simulink model "Locomotive_model"  (R2021a)
settings: Solver=ode23s  StartTime=0.0  StopTime=400  RelTol=1e-3
values from neighbouring files (symbols this model uses):
  B = T_friction/omega_b    (= 27.8481991909)    [Train_script.m]
  d = 1250*10^-3    (= 1.25)    [Train_script.m]
  I_motor = Pe_tot/sqrt(3)/V_motor/cos_fi    [Train_script.m]
  id_ref = psi_rd_ref./M    [Train_script.m]
  J = mass_tot*v_max^2/omega_max^2    (= 15228.5481732)    [Train_script.m]
  kp_O = par_reg_speed.Kp    [Train_script.m]
  kp_psi = par_reg_speed.Kp    [Train_script.m]
  kp_s = par_regi.Kp    [Train_script.m]
  Lks = X_lock_eq/(2*pi*50)    [Train_script.m]
  M = (X_noload_eq)/(2*pi*50)    [Train_script.m]
  mass_tot = 89*10^3+11*47*10^3+45*80+45*15    (= 610275)    [Train_script.m]
  pp = 2    [Train_script.m]
  psi_r_max = V_motor*sqrt(3)*0.8/(omega_b*pp)    [Train_script.m]
  psi_rd_ref = traction(:,2).*d/2.*tr./k    [Train_script.m]
  Rks = Rs_eq+Rr_eq    [Train_script.m]
  Rr_eq = Rr*Z    [Train_script.m]
  Rs_eq = Rs*Z    [Train_script.m]
  speed_ref = traction(:,1)    [Train_script.m]
  Ti_O = kp_O/ki_O    [Train_script.m]
  Ti_psi = kp_psi/ki_psi    [Train_script.m]
  Ti_s = kp_s/ki_s    [Train_script.m]
  tr = 23/91    (= 0.252747252747)    [Train_script.m]
  traction = [0 5.21669680807 10.1836330644 15.2754495965 20.3652465016 25.3331925714 30.1742387383 35.0162947187 40.1091210644 45.0750475071 50.0419837634 54.8850495574 ... (92 elements, 46x2)]    [Traction_e402B_online.mat]
  V_max = V_motor*sqrt(3)    [Train_script.m]
  V_motor = 1860    [Train_script.m]
undefined symbols (not defined in the file or in its folder): magnitude
libraries: simulink x7
settings Model: Creator=secch  LastModifiedBy=secch
settings SolverCC: ZeroCrossAlgorithm=Adaptive  AlgebraicLoopSolver=TrustRegion
settings DebuggingCC: IgnoredZcDiagnostic=none  SFMachineParentedDataDiag=warning

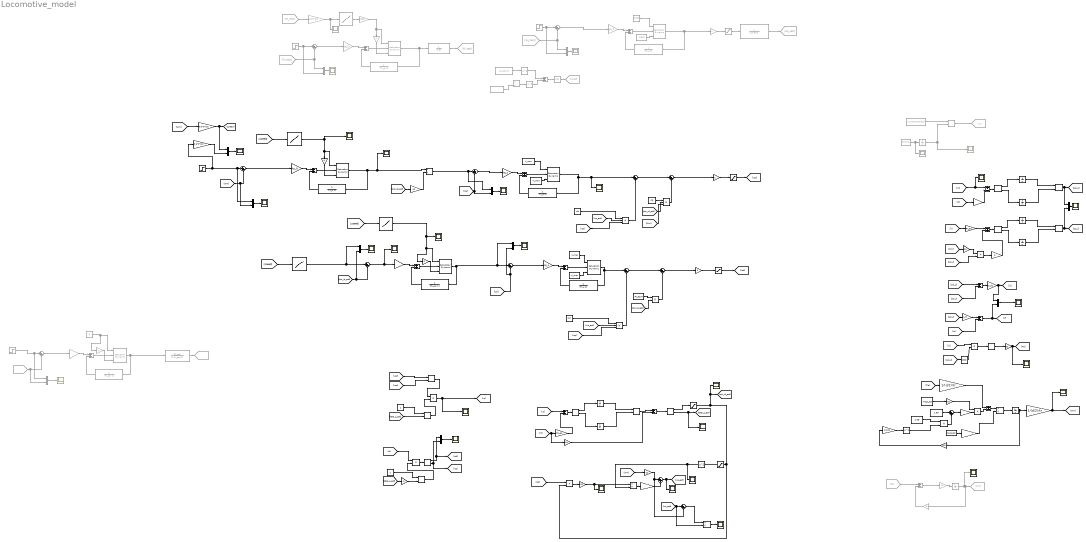
== system Locomotive_model ==
  note: Subsystem
  note: psi_rd_max
  1-D Lookup Table1 : Lookup_n-D  Commented=on  NumberOfTableDimensions=1  BreakpointsForDimension1=traction(:,1)  Table=traction(:,2)  InternalRulePriority=Speed  RndMeth=Simplest  InputSameDT=on
  1-D Lookup Table2 : Lookup_n-D  NumberOfTableDimensions=1  BreakpointsForDimension1=speed_ref  Table=psi_rd_ref  InternalRulePriority=Speed  RndMeth=Simplest  InputSameDT=on
  1-D Lookup Table3 : Lookup_n-D  NumberOfTableDimensions=1  BreakpointsForDimension1=traction(:,1)  Table=traction(:,2).*d/2.*tr  InternalRulePriority=Speed  RndMeth=Simplest  InputSameDT=on
  1-D Lookup Table4 : Lookup_n-D  NumberOfTableDimensions=1  BreakpointsForDimension1=speed_ref  Table=id_ref  InternalRulePriority=Speed  RndMeth=Simplest  InputSameDT=on
  Complex to Magnitude-Angle : ComplexToMagnitudeAngle
  Complex to Real-Imag{1..3,5} (4 alike) : ComplexToRealImag
  Complex to Real-Imag4 : ComplexToRealImag  Output=Imag
  Conj : Math  Operator=conj  SaturateOnIntegerOverflow=on
  Constant : Constant  Commented=on  Value=5
  Constant1 : Constant  Value=V_max
  Constant10 : Constant  Value=Rr_eq/M
  Constant11 : Constant  Value=-V_max
  Constant12 : Constant  Value=V_max
  Constant13 : Constant  Value=-V_max
  Constant14 : Constant  Commented=on  Value=V_motor*sqrt(3/2)
  Constant15 : Constant  Commented=on  Value=2000
  Constant16 : Constant
  Constant17 : Constant
  Constant18 : Constant  Commented=on  Value=-2000
  Constant2 : Constant  Value=2.05
  Constant21 : Constant  Commented=on  Value=pp*psi_r_max
  Constant22 : Constant  Commented=on  Value=I_motor*2
  Constant3 : Constant  Value=mass_tot
  Constant4 : Constant  Value=mass_tot
  Constant5 : Constant  Value=1.65
  Constant6 : Constant  Value=Lks
  Constant7 : Constant  Commented=on  Value=50*2*pi
  Constant8 : Constant  Value=pp
  Constant9 : Constant  Value=Lks
  Divide{,1..2,6} (4 alike) : Product  Inputs=*/
  Divide4 : Product  Commented=on  Inputs=*/
  From23 : From  Commented=on  GotoTag=isq_test
  From24 : From  Commented=on  GotoTag=W_test
  From25 : From  Commented=on  GotoTag=Te
  From26 : From  Commented=on  GotoTag=W_test
  From27 : From  Commented=on  GotoTag=psi_rd_test
  Gain1 : Gain
  Gain10 : Gain  Gain=kp_psi
  Gain11 : Gain  Gain=kp_s
  Gain12 : Gain  Gain=Rs_eq
  Gain13 : Gain  Gain=Rr_eq/pp
  Gain{14,18..19,23,42} (5 alike) : Gain  Gain=pp
  Gain15 : Gain  Gain=3.6*tr*d/2
  Gain16 : Gain  Gain=(1+0.075)
  Gain17 : Gain  Gain=Rs_eq
  Gain2 : Gain
  Gain20 : Gain  Gain=1/1000
  Gain21 : Gain  Gain=1i
  Gain22 : Gain  Gain=1/Lks
  Gain24 : Gain  Gain=1/M
  Gain25 : Gain  Gain=1/100
  Gain26 : Gain  Gain=Rr_eq
  Gain27 : Gain  Gain=1/(d/2)/tr
  Gain28 : Gain  Gain=3.6
  Gain29 : Gain  Gain=1/(d/2)/tr
  Gain3 : Gain  Gain=-1
  Gain30 : Gain  Gain=3.6*tr*d/2
  Gain31 : Gain  Commented=on  Gain=B
  Gain32 : Gain  Commented=on  Gain=1/J
  Gain33 : Gain  Commented=on  Gain=-1
  Gain34 : Gain  Commented=on  Gain=kp_O
  Gain35 : Gain  Commented=on  Gain=1000
  Gain36 : Gain  Commented=on  Gain=3.6*tr*d/2
  Gain38 : Gain  Commented=on  Gain=kp_s
  Gain39 : Gain  Commented=on
  Gain4 : Gain  Gain=Lks
  Gain40 : Gain  Commented=on  Gain=kp_psi
  Gain41 : Gain  Commented=on  Gain=-1
  Gain5 : Gain  Gain=9.8
  Gain6 : Gain  Gain=-1
  Gain7 : Gain  Gain=kp_O
  Gain8 : Gain  Gain=kp_s
  Gain9 : Gain  Gain=-1
  Goto13 : Goto  Commented=on  GotoTag=vs
  Goto14 : Goto  Commented=on  GotoTag=Wm
  Goto15 : Goto  Commented=on  GotoTag=W_test
  Goto16 : Goto  Commented=on  GotoTag=isq_test
  Goto17 : Goto  Commented=on  GotoTag=psi_rd_test
  Goto18 : Goto  Commented=on  GotoTag=id_ref
  Integrator{,1..6} (7 alike) : Integrator
  Integrator7 : Integrator  Commented=on
  Integrator8 : Integrator  Commented=on
  Magnitude Square : Math  Operator=magnitude^2  SignedPower=on  RndMeth=Zero  SaturateOnIntegerOverflow=on
  Magnitude-Angle to Complex2 : MagnitudeAngleToComplex
  Magnitude-Angle to Complex3 : MagnitudeAngleToComplex
  Magnitude-Angle to Complex4 : MagnitudeAngleToComplex  Commented=on
  Mux{,1..4,8..10} (8 alike) : Mux  Inputs=2
  Mux5 : Mux  Commented=on  Inputs=2
  Mux6 : Mux  Commented=on  Inputs=2
  Mux7 : Mux  Commented=on  Inputs=2
  Product{,3..7,10..11} (8 alike) : Product
  Product1 : Product  Inputs=3
  Product8 : Product  Inputs=3
  Product9 : Product  Inputs=3
  Real-Imag to Complex{1..4} (4 alike) : RealImagToComplex
  Saturation : Saturate  UpperLimit=4.2  LowerLimit=-4.2
  Saturation Dynamic{,1..3} (4 alike) : simulink/Discontinuities/Saturation Dynamic  OutMin=[]  OutMax=[]  OutDataTypeStr=Inherit: Same as second input  OutDataType=fixdt(1, 16)  OutScaling=2^-10  DoSatur=off
  Saturation Dynamic4 : simulink/Discontinuities/Saturation Dynamic  Commented=on  OutMin=[]  OutMax=[]  OutDataTypeStr=Inherit: Same as second input  OutDataType=fixdt(1, 16)  OutScaling=2^-10  DoSatur=off
  Saturation Dynamic5 : simulink/Discontinuities/Saturation Dynamic  Commented=on  OutMin=[]  OutMax=[]  OutDataTypeStr=Inherit: Same as second input  OutDataType=fixdt(1, 16)  OutScaling=2^-10  DoSatur=off
  Saturation Dynamic6 : simulink/Discontinuities/Saturation Dynamic  Commented=on  OutMin=[]  OutMax=[]  OutDataTypeStr=Inherit: Same as second input  OutDataType=fixdt(1, 16)  OutScaling=2^-10  DoSatur=off
  Saturation1 : Saturate  UpperLimit=V_max  LowerLimit=-V_max  LinearizeAsGain=off
  Saturation2 : Saturate  Commented=on  UpperLimit=20000  LowerLimit=-20000
  Saturation3 : Saturate  UpperLimit=V_max  LowerLimit=-V_max  LinearizeAsGain=off
  Saturation4 : Saturate  UpperLimit=8  LowerLimit=0.01
  Scope{,1..6,8..11,14..15,19..28} (23 alike) : Scope
  Scope{7,12..13,16..18} (6 alike) : Scope  Commented=on
  Square : Math  Operator=square  SaturateOnIntegerOverflow=on
  Square Root1 : Sqrt  Commented=on  SaturateOnIntegerOverflow=on
  Square3 : Math  Commented=on  Operator=square  SaturateOnIntegerOverflow=on
  Square4 : Math  Commented=on  Operator=square  SaturateOnIntegerOverflow=on
  Step : Step  Commented=on  After=350  SampleTime=0
  Step1 : Step  Commented=on  After=5000  SampleTime=0
  Step2 : Step  Commented=on  After=4  SampleTime=0
  Step3 : Step  Time=2  After=350  SampleTime=0
  Sum : Sum  Inputs=|++
  Sum1 : Sum  Inputs=|++
  Sum2 : Sum  Inputs=|+-
  Sum3 : Sum  Commented=on  Inputs=|+-
  Sum4 : Sum  Commented=on  Inputs=|+-
  Transfer Fcn : TransferFcn  Commented=on  Denominator=[J B]
  Transfer Fcn1 : TransferFcn  Commented=on  Denominator=[Ti_O 1]
  Transfer Fcn2 : TransferFcn  Commented=on  Denominator=[Ti_s 1]
  Transfer Fcn3 : TransferFcn  Commented=on  Denominator=[Ti_psi 1]
  Transfer Fcn4 : TransferFcn  Commented=on  Denominator=[Lks Rks]
  Transfer Fcn5 : TransferFcn  Denominator=[Ti_O 1]
  Transfer Fcn6 : TransferFcn  Denominator=[Ti_s 1]
  Transfer Fcn7 : TransferFcn  Denominator=[Ti_psi 1]
  Transfer Fcn8 : TransferFcn  Denominator=[Ti_s 1]
  Transfer Fcn9 : TransferFcn  Commented=on  Numerator=[Rr_eq]  Denominator=[1 Rr_eq/M]
  scorrimento : Scope
  sum{1..2,19..22} (6 alike) : Sum  Inputs=+-
  sum{6,10..14} (6 alike) : Sum  Inputs=|+-
  sum{15..18} (4 alike) : Sum
  sum23 : Sum  Commented=on  Inputs=|+-
  sum24 : Sum  Commented=on
  sum26 : Sum  Commented=on  Inputs=+-
  sum3 : Sum  Inputs=-+
  sum4 : Sum  Commented=on  Inputs=+-
  sum5 : Sum  Commented=on
  sum7 : Sum  Commented=on
  sum8 : Sum  Inputs=|++
  sum9 : Sum  Inputs=|++
  wires:
  sum9/1 -> Gain1/1
  sum14/1 -> Gain2/1
  [isd] -> Mux9/2, sum12/2
  1-D Lookup Table2/1 -> Mux10/1, sum10/1
  Saturation Dynamic2/1 -> Transfer Fcn7/1, Mux9/1, sum12/1
  Saturation Dynamic3/1 -> Transfer Fcn8/1, sum13/1
  [isq] -> Product9/3
  Product9/1 -> sum13/2
  Constant9/1 -> Product9/1
  [ws_est] -> Product9/2
  Constant10/1 -> Product10/1
  [psi_rd_est] -> Product10/2
  Product10/1 -> sum14/2
  sum13/1 -> sum14/1
  sum8/1 -> sum9/1
  Product8/1 -> sum9/2
  [Wm] -> Product8/3
  [psi_rd_est] -> Product8/2
  Constant8/1 -> Product8/1
  [ws_est] -> Product1/2
  Constant6/1 -> Product1/1
  Product1/1 -> sum8/2
  [isd] -> Product1/3
  Saturation Dynamic1/1 -> Scope26/1, sum8/1, Transfer Fcn6/1
  Saturation Dynamic/1 -> Divide6/1, Scope22/1, Transfer Fcn5/1
  [Wm] -> Mux/2, sum11/2
  [isq] -> sum6/2, Mux8/2
  Gain7/1 -> sum15/1
  sum15/1 -> Saturation Dynamic/2
  sum11/1 -> Gain7/1
  [speed] -> 1-D Lookup Table3/1
  Gain6/1 -> Saturation Dynamic/3
  Transfer Fcn5/1 -> sum15/2
  Transfer Fcn6/1 -> sum16/2
  Constant11/1 -> Saturation Dynamic1/3
  Constant1/1 -> Saturation Dynamic1/1
  sum6/1 -> Gain8/1
  sum16/1 -> Saturation Dynamic1/2
  Gain8/1 -> sum16/1
  Transfer Fcn7/1 -> sum17/2
  Gain9/1 -> Saturation Dynamic2/3
  1-D Lookup Table4/1 -> Saturation Dynamic2/1, Gain9/1, Scope28/1
  sum10/1 -> Scope27/1, Gain10/1
  sum17/1 -> Saturation Dynamic2/2
  Gain10/1 -> sum17/1
  Gain11/1 -> sum18/1
  sum18/1 -> Saturation Dynamic3/2
  sum12/1 -> Gain11/1
  Constant12/1 -> Saturation Dynamic3/1
  Constant13/1 -> Saturation Dynamic3/3
  Transfer Fcn8/1 -> sum18/2
  Integrator1/1 -> Real-Imag to Complex3/2
  Integrator/1 -> Real-Imag to Complex3/1
  sum19/1 -> Complex to Real-Imag2/1
  Complex to Real-Imag2/1 -> Integrator/1
  Gain12/1 -> sum19/2
  [vs] -> sum19/1
  [is] -> Gain12/1, Gain4/1
  Complex to Real-Imag2/2 -> Integrator1/1
  Real-Imag to Complex3/1 -> sum20/1
  Gain4/1 -> sum20/2
  sum20/1 -> Complex to Magnitude-Angle/1
  Complex to Magnitude-Angle/2 -> Scope8/1, [teta_s_est]
  Saturation/1 -> Square/1
  Divide/1 -> Gain13/1
  Gain13/1 -> Sum/2
  [Wm] -> Gain14/1
  Gain14/1 -> Sum/1, Sum2/2
  Sum/1 -> Scope11/1, [ws_est]
  Product/1 -> Gain19/1
  [isq] -> Product/1
  Gain19/1 -> Scope15/1, Divide/1
  [teta_s_est] -> Magnitude-Angle to Complex2/2
  Magnitude-Angle to Complex2/1 -> Product3/2
  Constant16/1 -> Magnitude-Angle to Complex2/1
  Constant17/1 -> Magnitude-Angle to Complex3/1
  [teta_s_est] -> Gain3/1
  Gain2/1 -> Saturation3/1
  Gain1/1 -> Saturation1/1
  [Wm] -> Gain15/1
  Gain15/1 -> Mux3/1, [speed]
  Complex to Real-Imag1/1 -> [isd], Mux4/1
  Complex to Real-Imag1/2 -> [isq], Mux4/2
  Product4/1 -> Complex to Real-Imag1/1
  [is] -> Product4/1
  Gain3/1 -> Magnitude-Angle to Complex3/2
  Magnitude-Angle to Complex3/1 -> Product4/2
  Divide1/1 -> Integrator5/1
  Gain16/1 -> Divide1/2
  sum2/1 -> Divide1/1
  Gain29/1 -> sum2/1
  [Te] -> Gain29/1
  Gain5/1 -> Product7/1
  Product7/1 -> sum2/2
  Constant3/1 -> Gain5/1
  Magnitude Square/1 -> Product6/2
  Gain28/1 -> Gain25/1
  Integrator5/1 -> Gain28/1, Gain27/1
  Gain27/1 -> Scope3/1, [Wm]
  Gain25/1 -> Magnitude Square/1
  Constant2/1 -> Product6/1
  Product6/1 -> Sum1/2
  Constant5/1 -> Sum1/1
  Constant4/1 -> Gain16/1
  Gain23/1 -> Scope1/1, [Te]
  [is] -> Gain17/1
  Real-Imag to Complex2/1 -> Mux1/1, [psi_s]
  [is] -> Product11/1
  sum1/1 -> Complex to Real-Imag5/1
  Gain21/1 -> sum3/2
  [psi_r] -> Product5/2
  [psi_s] -> sum21/1
  Product11/1 -> Complex to Real-Imag4/1
  Gain26/1 -> sum3/1
  [Wm] -> Gain18/1
  Complex to Real-Imag3/2 -> Integrator3/1
  Integrator2/1 -> Real-Imag to Complex4/1
  Product5/1 -> Gain21/1
  sum3/1 -> Complex to Real-Imag3/1
  Integrator6/1 -> Real-Imag to Complex2/2
  Gain17/1 -> sum1/2
  [is] -> sum22/2
  [psi_r] -> sum21/2
  Integrator4/1 -> Real-Imag to Complex2/1
  Gain24/1 -> sum22/1
  Complex to Real-Imag4/1 -> Gain23/1
  [psi_s] -> Conj/1
  Complex to Real-Imag5/1 -> Integrator4/1
  [vs] -> Scope5/1, sum1/1
  Conj/1 -> Product11/2
  sum21/1 -> Gain22/1
  Real-Imag to Complex4/1 -> Mux1/2, [psi_r]
  Complex to Real-Imag5/2 -> Integrator6/1
  Integrator3/1 -> Real-Imag to Complex4/2
  [ir] -> Gain26/1
  [psi_r] -> Gain24/1
  Complex to Real-Imag3/1 -> Integrator2/1
  Gain22/1 -> Mux2/1, [is]
  sum22/1 -> Mux2/2, [ir]
  Gain18/1 -> Product5/1
  [psi_rd_est] -> Mux10/2, sum10/2
  Mux/1 -> Scope/1
  Square/1 -> Scope14/1, Divide/2
  Mux1/1 -> Scope2/1
  Mux2/1 -> Scope4/1
  Sum1/1 -> Gain20/1
  Gain20/1 -> Product7/2
  Step3/1 -> Gain30/1, Mux/1, sum11/1
  Mux3/1 -> Scope6/1
  Gain30/1 -> Mux3/2
  Mux4/1 -> Scope9/1
  Magnitude-Angle to Complex4/1 -> Goto13/1
  Gain31/1 -> sum4/2
  From25/1 -> sum4/1
  sum4/1 -> Gain32/1
  Gain32/1 -> Integrator7/1
  Integrator7/1 -> Scope10/1, Gain31/1, Goto14/1
  Constant7/1 -> Scope16/1, Integrator8/1
  Constant14/1 -> Magnitude-Angle to Complex4/1
  Integrator8/1 -> Scope13/1, Magnitude-Angle to Complex4/2
  Sum2/1 -> Divide2/1
  [ws_est] -> Divide2/2, Sum2/1
  Divide2/1 -> scorrimento/1
  [vsq] -> Real-Imag to Complex1/2
  [vsd] -> Real-Imag to Complex1/1
  1-D Lookup Table1/1 -> Gain35/1
  Transfer Fcn1/1 -> sum5/2
  Gain33/1 -> Saturation Dynamic4/3
  Gain36/1 -> Scope12/1, 1-D Lookup Table1/1
  sum5/1 -> Saturation Dynamic4/2
  Gain34/1 -> sum5/1
  Saturation Dynamic4/1 -> Transfer Fcn/1, Transfer Fcn1/1
  Sum3/1 -> Gain34/1
  Step/1 -> Mux5/2, Sum3/1
  Mux5/1 -> Scope7/1
  From24/1 -> Mux5/1, Sum3/2
  Transfer Fcn/1 -> Goto15/1
  From26/1 -> Gain36/1
  Gain35/1 -> Gain33/1, Saturation Dynamic4/1
  Gain38/1 -> sum7/1
  sum7/1 -> Saturation Dynamic5/2
  Constant15/1 -> Saturation Dynamic5/1
  Constant18/1 -> Saturation Dynamic5/3
  Transfer Fcn2/1 -> sum7/2
  From23/1 -> Sum4/2, Mux6/1
  Mux6/1 -> Scope17/1
  Step1/1 -> Sum4/1, Mux6/2
  Sum4/1 -> Gain38/1
  Gain39/1 -> Saturation2/1
  Saturation2/1 -> Transfer Fcn4/1
  Saturation Dynamic5/1 -> Gain39/1, Transfer Fcn2/1
  Transfer Fcn4/1 -> Goto16/1
  From27/1 -> Mux7/2, sum23/2
  Gain40/1 -> sum24/1
  sum24/1 -> Saturation Dynamic6/2
  sum23/1 -> Gain40/1
  Constant/1 -> Gain41/1, Saturation Dynamic6/1
  Gain41/1 -> Saturation Dynamic6/3
  Transfer Fcn3/1 -> sum24/2
  Saturation Dynamic6/1 -> Transfer Fcn9/1, Transfer Fcn3/1
  Transfer Fcn9/1 -> Goto17/1
  Step2/1 -> Mux7/1, sum23/1
  Mux7/1 -> Scope18/1
  Complex to Magnitude-Angle/1 -> Saturation4/1
  Mux8/1 -> Scope23/1
  Mux9/1 -> Scope24/1
  Mux10/1 -> Scope25/1
  Real-Imag to Complex1/1 -> Product3/1
  Product3/1 -> [vs], Scope19/1
  Saturation1/1 -> [vsq]
  Saturation3/1 -> [vsd]
  Saturation4/1 -> Scope20/1, [psi_rd_est], Saturation/1, Product/2
  Divide6/1 -> Mux8/1, sum6/1
  Gain42/1 -> Divide6/2
  [psi_rd_est] -> Gain42/1
  1-D Lookup Table3/1 -> Saturation Dynamic/1, Gain6/1, Scope21/1
  [speed] -> 1-D Lookup Table2/1
  [speed] -> 1-D Lookup Table4/1
  Constant22/1 -> Square4/1
  Square Root1/1 -> Goto18/1
  sum26/1 -> Square Root1/1
  Square4/1 -> sum26/1
  Square3/1 -> sum26/2
  Divide4/1 -> Square3/1
  Constant21/1 -> Divide4/2
